simulink model "Testing"  (R2023b)
settings: Solver=FixedStepAuto  StartTime=0.0  StopTime=10.0  RelTol=1e-3
settings Model: Creator=tlgwo  LastModifiedBy=tlgwo
settings OptimizationCC: BlockReduction=off  ConditionallyExecuteInputs=off

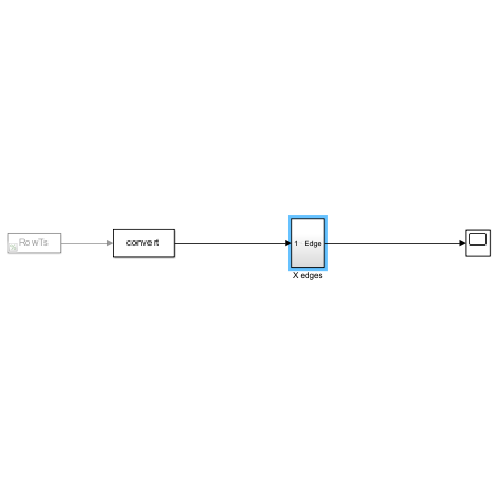
[thumbnail: Simulink's stored preview of the top-level diagram]
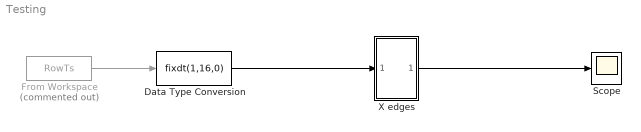
== system Testing ==
  Data Type Conversion : DataTypeConversion  OutDataTypeStr=fixdt(1,16,0)  SaturateOnIntegerOverflow=off  RndMeth=Floor
  From Workspace : FromWorkspace  Commented=on  VariableName=RowTs  SampleTime=1
  Scope : Scope
  X edges : Subsystem
  wires:
  From Workspace/1 -> Data Type Conversion/1
  X edges/1(Edge) -> Scope/1
  Data Type Conversion/1 -> X edges/1(In1)

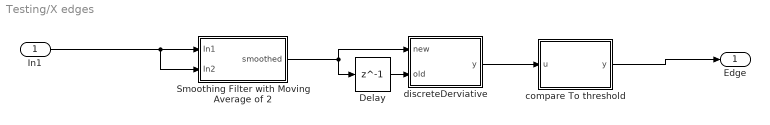
== system Testing/X edges ==
  In1 : Inport
  Delay : Delay  DelayLength=1
  Smoothing Filter with Moving Average of 2 : Subsystem
  compare To threshold : MATLAB Function  TreatAsAtomicUnit=on
  discreteDerviative : MATLAB Function  TreatAsAtomicUnit=on
  Edge : Outport
  wires:
  In1/1 -> Smoothing Filter with Moving Average of 2/2(In2), Smoothing Filter with Moving Average of 2/1(In1)
  compare To threshold/1(y) -> Edge/1
  Smoothing Filter with Moving Average of 2/1(smoothed) -> discreteDerviative/1(new), Delay/1
  Delay/1 -> discreteDerviative/2(old)
  discreteDerviative/1(y) -> compare To threshold/1(u)

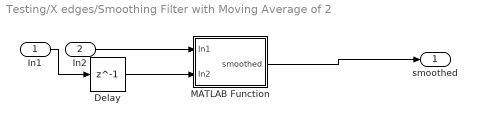
== system Testing/X edges/Smoothing Filter with Moving Average of 2 ==
  In1 : Inport
  In2 : Inport  Port=2
  Delay : Delay  DelayLength=1
  MATLAB Function : MATLAB Function  TreatAsAtomicUnit=on
  smoothed : Outport
  wires:
  Delay/1 -> MATLAB Function/2(In2)
  In2/1 -> MATLAB Function/1(In1)
  MATLAB Function/1(smoothed) -> smoothed/1
  In1/1 -> Delay/1

== matlab function Testing/X edges/Smoothing Filter with Moving Average of 2/MATLAB Function ==
  data: In1 input; smoothed output; In2 input
function smoothed = fcn(In1,In2)

smoothed = (In1 + In2);

== matlab function Testing/X edges/discreteDerviative ==
  data: new input; old input; y output
function y = fcn(new, old)

y = new - old;

== matlab function Testing/X edges/compare To threshold ==
  data: u input; y output
function y = fcn(u)

    if (abs(u) > 10);
        y = 1;
    else
        y = 0;
    end
